simulink model "BLDC_Motor_subsystem"  (R2020b)
settings: Solver=VariableStepAuto  StartTime=0.0  StopTime=10.0  RelTol=1e-3
model workspace (MAT data in the model file):
  den = [0.0001 0.014]
  den1 = [0.0002 0.004586]
  ke = 0.0275
  kt = 0.0275
  num = 1
settings Model: Creator=user  LastModifiedBy=user
settings DataIOCC: SaveOutput=off  SaveTime=off

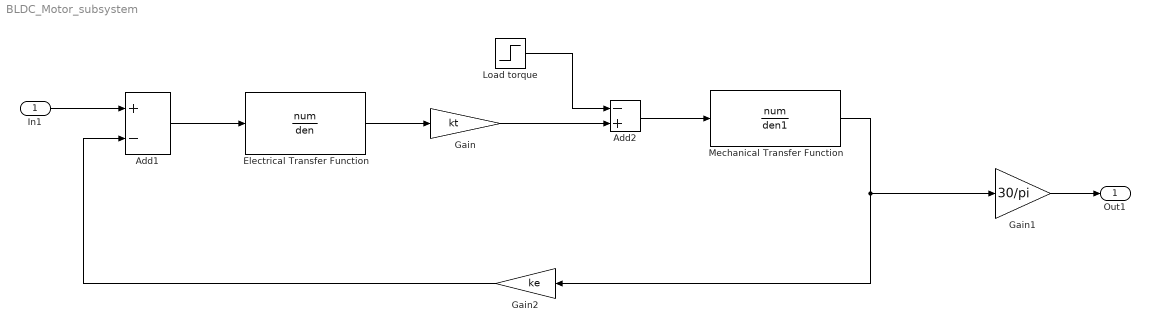
== system BLDC_Motor_subsystem ==
  In1 : Inport  OutDataTypeStr=double  PortDimensions=1  SampleTime=0
  Add1 : Sum  Inputs=+-
  Add2 : Sum  Inputs=-+
  Electrical Transfer Function : TransferFcn  Numerator=num  Denominator=den
  Gain : Gain  Gain=kt
  Gain1 : Gain  Gain=30/pi
  Gain2 : Gain  Gain=ke
  Load torque : Step  SampleTime=0
  Mechanical Transfer Function : TransferFcn  Numerator=num  Denominator=den1
  Out1 : Outport  OutDataTypeStr=double  PortDimensions=1  SampleTime=0
  wires:
  Add1/1 -> Electrical Transfer Function/1
  Gain1/1 -> Out1/1
  Electrical Transfer Function/1 -> Gain/1
  Mechanical Transfer Function/1 -> Gain1/1, Gain2/1
  Gain/1 -> Add2/2
  In1/1 -> Add1/1
  Add2/1 -> Mechanical Transfer Function/1
  Load torque/1 -> Add2/1
  Gain2/1 -> Add1/2
